simulink model "BMS_Status_AutoBuild"  (R2026a)
settings: Solver=VariableStepAuto
settings Model: Creator=tastytaco  LastModifiedBy=tastytaco

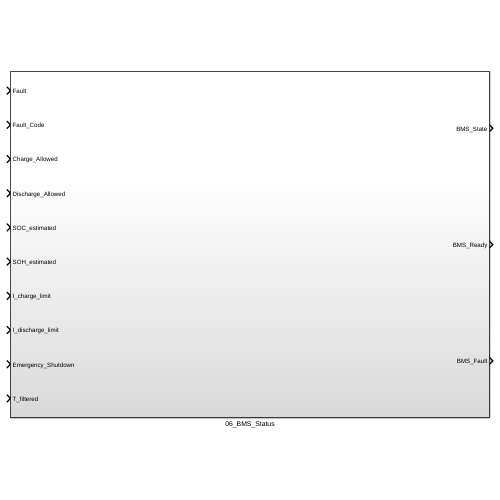
[thumbnail: Simulink's stored preview of the top-level diagram]
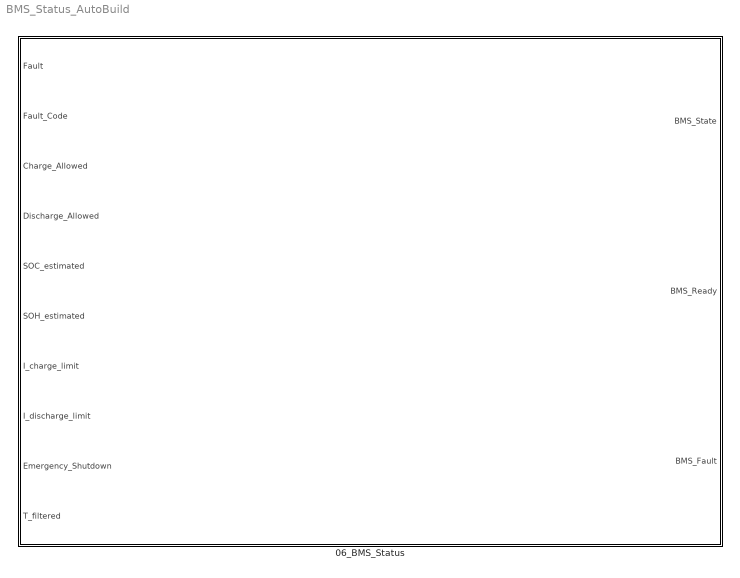
== system BMS_Status_AutoBuild ==
  06_BMS_Status : Subsystem

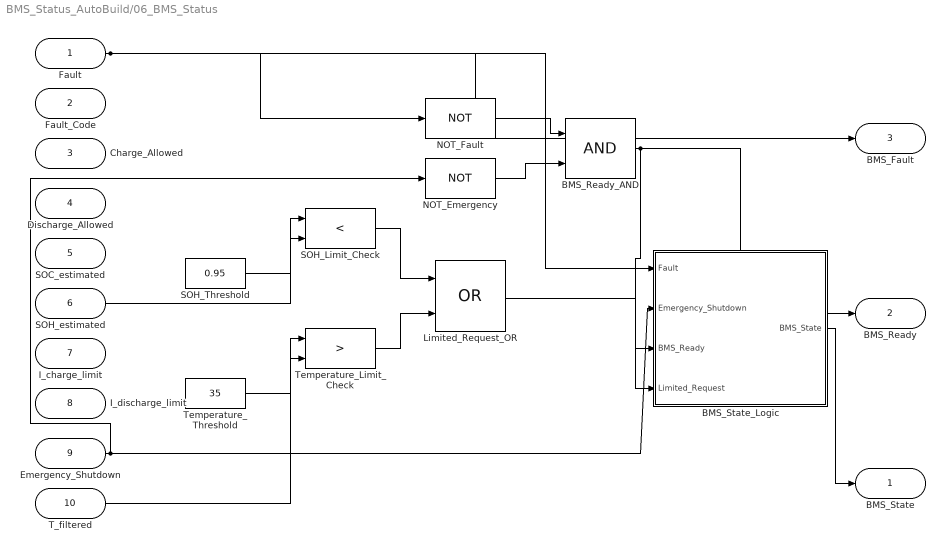
== system BMS_Status_AutoBuild/06_BMS_Status ==
  Fault : Inport
  Fault_Code : Inport  Port=2
  Charge_Allowed : Inport  Port=3
  Discharge_Allowed : Inport  Port=4
  SOC_estimated : Inport  Port=5
  SOH_estimated : Inport  Port=6
  I_charge_limit : Inport  Port=7
  I_discharge_limit : Inport  Port=8
  Emergency_Shutdown : Inport  Port=9
  T_filtered : Inport  Port=10
  BMS_Ready_AND : Logic  AllPortsSameDT=off  OutDataTypeStr=boolean
  BMS_State_Logic : MATLAB Function  TreatAsAtomicUnit=on
  Limited_Request_OR : Logic  Operator=OR  AllPortsSameDT=off  OutDataTypeStr=boolean
  NOT_Emergency : Logic  Operator=NOT  AllPortsSameDT=off  OutDataTypeStr=boolean
  NOT_Fault : Logic  Operator=NOT  AllPortsSameDT=off  OutDataTypeStr=boolean
  SOH_Limit_Check : RelationalOperator  Operator=<  OutDataTypeStr=boolean  RndMeth=Simplest  InputSameDT=off
  SOH_Threshold : Constant  Value=0.95
  Temperature_Limit_Check : RelationalOperator  Operator=>  OutDataTypeStr=boolean  RndMeth=Simplest  InputSameDT=off
  Temperature_Threshold : Constant  Value=35
  BMS_State : Outport
  BMS_Ready : Outport  Port=2
  BMS_Fault : Outport  Port=3
  wires:
  ? -> ?
  Fault/1 -> BMS_Fault/1, NOT_Fault/1, BMS_State_Logic/1(Fault)
  SOH_estimated/1 -> SOH_Limit_Check/1
  SOH_Threshold/1 -> SOH_Limit_Check/2
  T_filtered/1 -> Temperature_Limit_Check/1
  Temperature_Threshold/1 -> Temperature_Limit_Check/2
  SOH_Limit_Check/1 -> Limited_Request_OR/1
  Temperature_Limit_Check/1 -> Limited_Request_OR/2
  Emergency_Shutdown/1 -> NOT_Emergency/1, BMS_State_Logic/2(Emergency_Shutdown)
  NOT_Fault/1 -> BMS_Ready_AND/1
  NOT_Emergency/1 -> BMS_Ready_AND/2
  BMS_Ready_AND/1 -> BMS_Ready/1, BMS_State_Logic/3(BMS_Ready)
  Limited_Request_OR/1 -> BMS_State_Logic/4(Limited_Request)
  BMS_State_Logic/1(BMS_State) -> BMS_State/1

== matlab function BMS_Status_AutoBuild/06_BMS_Status/BMS_State_Logic ==
  data: Fault input; BMS_State output; Emergency_Shutdown input; BMS_Ready input; Limited_Request input
function BMS_State = fcn(Fault, Emergency_Shutdown, BMS_Ready, Limited_Request)

% BMS State Codes
% 0 = INIT
% 1 = NORMAL
% 2 = LIMITED
% 3 = FAULT
% 4 = SHUTDOWN

% Highest priority: Emergency Shutdown
if Emergency_Shutdown
    BMS_State = 4;

% Protection fault
elseif Fault
    BMS_State = 3;

% BMS not ready
elseif ~BMS_Ready
    BMS_State = 0;

% Battery operating under limitation
elseif Limited_Request
    BMS_State = 2;

% Normal operation
else
    BMS_State = 1;
end

end
